simulink model "GFLIB_ControllerPIrAW_BAM_F16"  (Simulink 8.3)
settings: Solver=ode45  StartTime=0.0  StopTime=10.0  RelTol=1e-3
undefined symbols (not defined in the file): f16CC1, f16CC2, u16NShift
settings Model: Creator=B17364  LastModifiedBy=B17364
settings DataIOCC: SignalLoggingSaveFormat=Dataset
settings DebuggingCC: UnderspecifiedInitializationDetection=Simplified  StateNameClashWarn=none
settings GRTTargetCC: CombineOutputUpdateFcns=on  GRTInterface=off

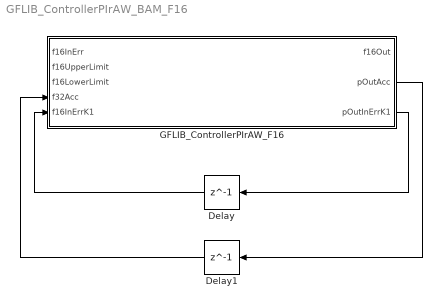
== system GFLIB_ControllerPIrAW_BAM_F16 ==
  Delay : Delay  DelayLength=1  InitialCondition=0
  Delay1 : Delay  DelayLength=1  InitialCondition=0
  GFLIB_ControllerPIrAW_F16 : Subsystem  mask(GFLIB_ControllerPIrAW_F16){f16CC1=f16CC1, f16CC2=f16CC2, u16NShift=u16NShift}
      mask help: Bit accurate model of reccurent form PI controller with anti-windup. All parameters as well as input and output are 16-bit integers except for u16NShift parameter which is 16-bit unsigned integer.
      mask init:
      | pos = get_param(gcb, 'Position');width = pos(3) - pos(1); height = pos(4) - pos(2);tX=width/2;tY=height*0.9;
      mask Display: color('black');port_label('input',1,'f16InErr');port_label('input',2,'f16UpperLimit');port_label('input',3,'f16LowerLimit');port_label('input',4,'f32Acc');port_label('input',5,'f16InErrK1');port_label('output',1,'f16Out');port_label('output',2,'pOutAcc');port_label('output',3,'pOutInErrK1');color('black');disp('GFLIB_ControllerPIrAW_F16');color('blue');text(tX,tY, 'BAM', 'horizontalAlignment', 'center');
  wires:
  GFLIB_ControllerPIrAW_F16/3(pOutInErrK1) -> Delay/1
  GFLIB_ControllerPIrAW_F16/2(pOutAcc) -> Delay1/1
  Delay/1 -> GFLIB_ControllerPIrAW_F16/5(f16InErrK1)
  Delay1/1 -> GFLIB_ControllerPIrAW_F16/4(f32Acc)

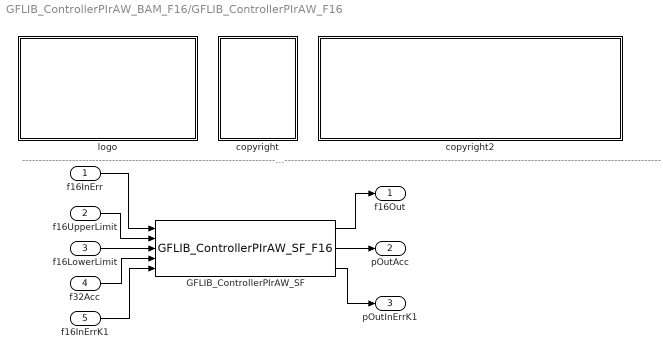
== system GFLIB_ControllerPIrAW_BAM_F16/GFLIB_ControllerPIrAW_F16 ==
  note: ---------------------------------------------------------------------------------------------------------------------------------------------------------------------------------------------------
  f16InErr : Inport
  f16UpperLimit : Inport  Port=2
  f16LowerLimit : Inport  Port=3
  f32Acc : Inport  Port=4
  f16InErrK1 : Inport  Port=5
  GFLIB_ControllerPIrAW_SF : S-Function  FunctionName=GFLIB_ControllerPIrAW_SF_F16  Parameters=f16CC1,f16CC2,u16NShift  EnableBusSupport=off
  copyright : Subsystem
      mask Display: text(10,90,'FILE:');text(10,75,'DESRIPTION:');text(10,60,'COPYRIGHT:');text(10,45,'VERSION:');text(10,30,'DATE:')
  copyright2 : Subsystem
      mask Display: text(10,90,'GFLIB_ControllerPIrAW_BAM_F16.mdl');text(10,75,'Recurrent form of a standard PI controller with implemented anti-windup functionality.');text(10,60,'Freescale');text(10,45,'0.1');text(10,30,'12-Jun-2015');
  logo : Subsystem
      mask Display: image(imread('logo.jpg'))
  f16Out : Outport
  pOutAcc : Outport  Port=2
  pOutInErrK1 : Outport  Port=3
  wires:
  f16InErr/1 -> GFLIB_ControllerPIrAW_SF/1
  f16UpperLimit/1 -> GFLIB_ControllerPIrAW_SF/2
  f16LowerLimit/1 -> GFLIB_ControllerPIrAW_SF/3
  f32Acc/1 -> GFLIB_ControllerPIrAW_SF/4
  f16InErrK1/1 -> GFLIB_ControllerPIrAW_SF/5
  GFLIB_ControllerPIrAW_SF/1 -> f16Out/1
  GFLIB_ControllerPIrAW_SF/2 -> pOutAcc/1
  GFLIB_ControllerPIrAW_SF/3 -> pOutInErrK1/1

== system GFLIB_ControllerPIrAW_BAM_F16/GFLIB_ControllerPIrAW_F16/copyright ==

== system GFLIB_ControllerPIrAW_BAM_F16/GFLIB_ControllerPIrAW_F16/copyright2 ==

== system GFLIB_ControllerPIrAW_BAM_F16/GFLIB_ControllerPIrAW_F16/logo ==
